simulink model "OnlyCombSlipTire"  (R2021b)
settings: Solver=ode4  StartTime=0.0  StopTime=1  FixedStep=0.001  RelTol=1e-3
values from neighbouring files (symbols this model uses):
  g = 9.80665    [VehicleParamsFEM20.m]    (also in VehicleParamsFEM20_Gear17.m; VehicleParamsFEM21.m)
  mu_tire_F = 0.587-0.587+0.55    (= 0.55)    [VehicleParamsFEM20.m]    (also in VehicleParamsFEM20_Gear17.m; VehicleParamsFEM21.m)
  W0_F = M*WBf/2    (= 62.4)    [VehicleParamsFEM20.m]    (also in VehicleParamsFEM20_Gear17.m; VehicleParamsFEM21.m)
libraries: simulink x2
settings Model: Creator=tsuyoshi  LastModifiedBy=tsuyoshi

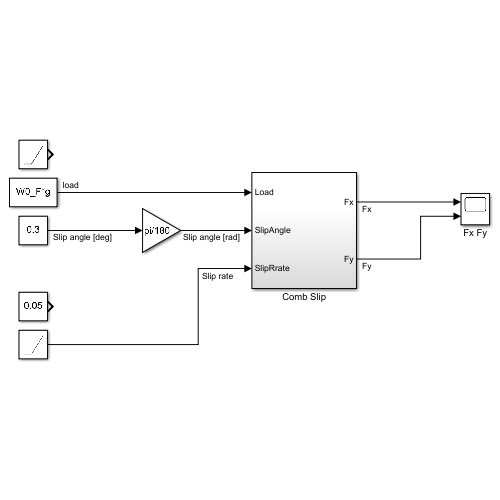
[thumbnail: Simulink's stored preview of the top-level diagram]
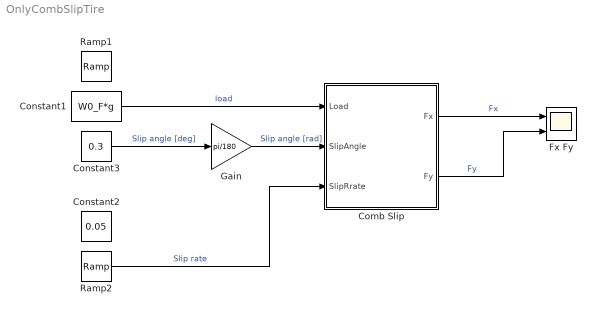
== system OnlyCombSlipTire ==
  Comb Slip : Subsystem
  Constant1 : Constant  Value=W0_F*g
  Constant2 : Constant  Value=0.05
  Constant3 : Constant  Value=0.3
  Fx Fy : Scope  NumInputPorts=2
  Gain : Gain  Gain=pi/180
  Ramp1 : simulink/Sources/Ramp  slope=W0_F*g  start=0  InitialOutput=0
  Ramp2 : simulink/Sources/Ramp  slope=1  start=0  InitialOutput=0
  wires:
  Ramp2/1 -> Comb Slip/3(SlipRrate)  "Slip rate"
  Constant1/1 -> Comb Slip/1(Load)  "load"
  Comb Slip/1(Fx) -> Fx Fy/1  "Fx"
  Comb Slip/2(Fy) -> Fx Fy/2  "Fy"
  Gain/1 -> Comb Slip/2(SlipAngle)  "Slip angle [rad]"
  Constant3/1 -> Gain/1  "Slip angle [deg]"

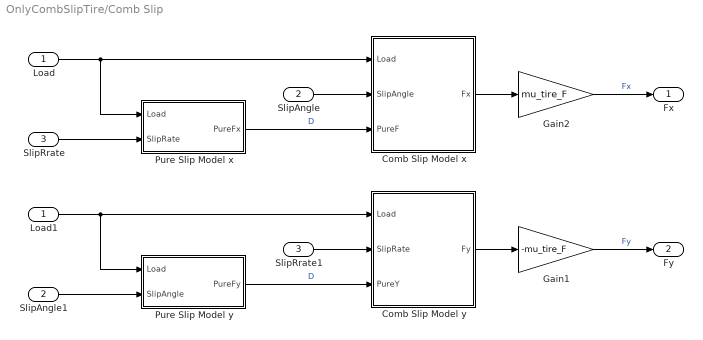
== system OnlyCombSlipTire/Comb Slip ==
  Load : Inport
  SlipAngle : Inport  Port=2
  SlipRrate : Inport  Port=3
  Comb Slip Model x : MATLAB Function  TreatAsAtomicUnit=on
  Comb Slip Model y : MATLAB Function  TreatAsAtomicUnit=on
  Gain1 : Gain  Gain=-mu_tire_F
  Gain2 : Gain  Gain=mu_tire_F
  Load1 : InportShadow
  Pure Slip Model x : MATLAB Function  TreatAsAtomicUnit=on
  Pure Slip Model y : MATLAB Function  TreatAsAtomicUnit=on
  SlipAngle1 : InportShadow  Port=2
  SlipRrate1 : InportShadow  Port=3
  Fx : Outport
  Fy : Outport  Port=2
  wires:
  Load/1 -> Pure Slip Model x/1(Load), Comb Slip Model x/1(Load)
  Pure Slip Model x/1(PureFx) -> Comb Slip Model x/3(PureF)  "D"
  SlipRrate/1 -> Pure Slip Model x/2(SlipRate)
  SlipAngle/1 -> Comb Slip Model x/2(SlipAngle)
  Comb Slip Model x/1(Fx) -> Gain2/1
  Gain2/1 -> Fx/1  "Fx"
  Gain1/1 -> Fy/1  "Fy"
  Comb Slip Model y/1(Fy) -> Gain1/1
  SlipAngle1/1 -> Pure Slip Model y/2(SlipAngle)
  SlipRrate1/1 -> Comb Slip Model y/2(SlipRate)
  Pure Slip Model y/1(PureFy) -> Comb Slip Model y/3(PureY)  "D"
  Load1/1 -> Comb Slip Model y/1(Load), Pure Slip Model y/1(Load)

== matlab function OnlyCombSlipTire/Comb Slip/Comb Slip Model x ==
  data: Load input; Fx output; SlipAngle input; agx_f parameter; PureF input
function Fx = fcn(Load, SlipAngle, agx_f, PureF)
    C = agx_f(1);
    D = PureF;
    E = Load*agx_f(4) + agx_f(5);
    B = agx_f(2)*sin(2*atan(Load/agx_f(3)))/(D*C);
    Fx = D*cos(C*atan(B*SlipAngle-E*(B*SlipAngle-atan(B*SlipAngle))));
end

== matlab function OnlyCombSlipTire/Comb Slip/Pure Slip Model x ==
  data: Load input; PureFx output; SlipRate input; afx_f parameter
function PureFx = fcn(Load, SlipRate, afx_f)
    C = afx_f(1);
    D = (Load*afx_f(2) + afx_f(3))*Load;
    E = Load*afx_f(6) + afx_f(7);
    B = afx_f(4)*sin(2*atan(Load/afx_f(5)))/(D*C);
    PureFx = D*sin(C*atan(B*SlipRate-E*(B*SlipRate-atan(B*SlipRate))));
end

== matlab function OnlyCombSlipTire/Comb Slip/Comb Slip Model y ==
  data: Load input; Fy output; SlipRate input; agy_f parameter; PureY input
function Fy = fcn(Load, SlipRate, agy_f, PureY)
    C = agy_f(1);
    D = PureY;
    E = Load*agy_f(4) + agy_f(5);
    B = agy_f(2)*sin(2*atan(Load/agy_f(3)))/(D*C);
    Fy = D*cos(C*atan(B*SlipRate-E*(B*SlipRate-atan(B*SlipRate))));
end

== matlab function OnlyCombSlipTire/Comb Slip/Pure Slip Model y ==
  data: Load input; PureFy output; SlipAngle input; a_f parameter
function PureFy = fcn(Load, SlipAngle, a_f)
    C = a_f(1);
    D = (Load*a_f(2) + a_f(3))*Load;
    E = Load*a_f(6) + a_f(7);
    B = a_f(4)*sin(2*atan(Load/a_f(5)))/(D*C);
    PureFy = D*sin(C*atan(B*SlipAngle-E*(B*SlipAngle-atan(B*SlipAngle))));
end
